simulink model "SVPWM_2L_Current_Loop"  (R2025a)
settings: Solver=VariableStepAuto  StartTime=0.0  StopTime=1  RelTol=1e-3
undefined symbols (not defined in the file): gTs
libraries: spsIGBTDiodeLib x6, spsVoltageMeasurementLib x6, spsACVoltageSourceLib x3, spsCurrentMeasurementLib x3, spsSeriesRLCBranchLib x3, simulink x1, spsDCVoltageSourceLib x1, sps_lib x1
settings Model: Creator=jicai  LastModifiedBy=jicai

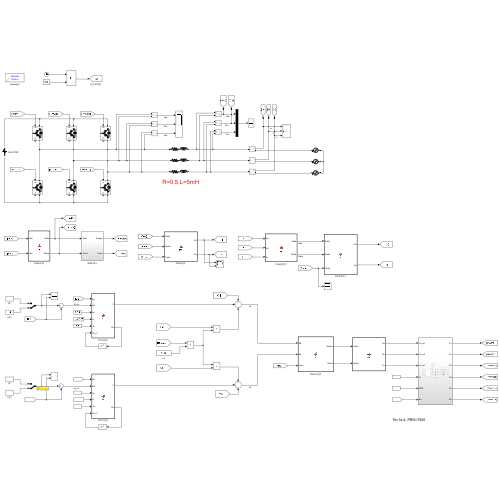
[thumbnail: Simulink's stored preview of the top-level diagram]
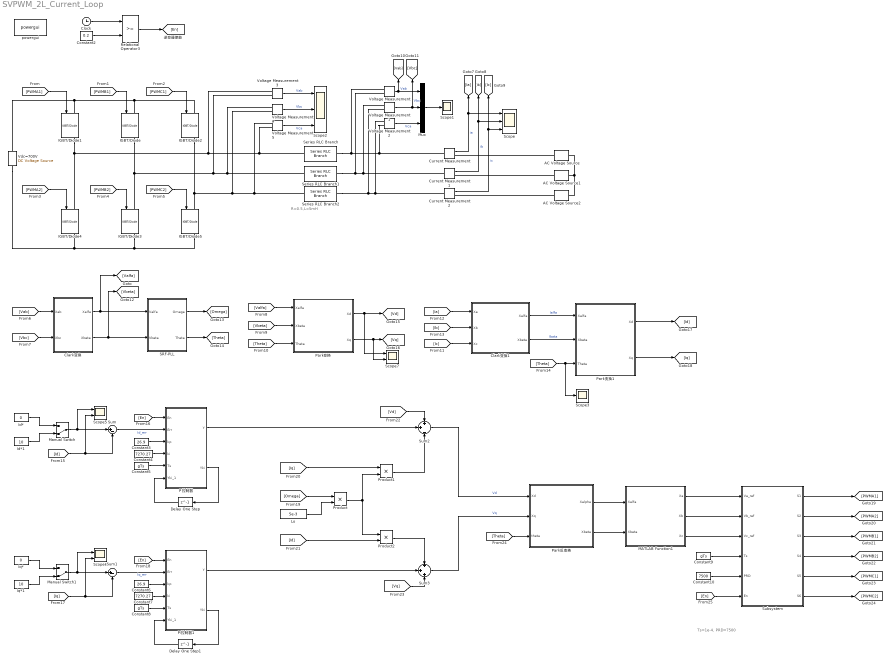
== system SVPWM_2L_Current_Loop ==
  note: R=0.5,L=5mH
  note: Ts=1e-4, PRD=7500
  AC Voltage Source : spsACVoltageSourceLib/AC Voltage Source  Amplitude=311  Phase=0  Frequency=50  SampleTime=1e-4  Measurements=None  BusType=swing  Pref=10e3  Qref=0  Qmin=-inf  Qmax=+inf
  AC Voltage Source1 : spsACVoltageSourceLib/AC Voltage Source  Amplitude=311  Phase=-120  Frequency=50  SampleTime=1e-4  Measurements=None  BusType=swing  Pref=10e3  Qref=0  Qmin=-inf  Qmax=+inf
  AC Voltage Source2 : spsACVoltageSourceLib/AC Voltage Source  Amplitude=311  Phase=120  Frequency=50  SampleTime=1e-4  Measurements=None  BusType=swing  Pref=10e3  Qref=0  Qmin=-inf  Qmax=+inf
  Clark变换 : MATLAB Function  TreatAsAtomicUnit=on
  Clark变换1 : MATLAB Function  TreatAsAtomicUnit=on
  Clock : Clock
  Constant10 : Constant  Value=7500
  Constant2 : Constant  Value=0.2
  Constant3 : Constant  Value=26.9
  Constant4 : Constant  Value=7270.27
  Constant5 : Constant  Value=gTs
  Constant6 : Constant  Value=26.9
  Constant7 : Constant  Value=7270.27
  Constant8 : Constant  Value=gTs
  Constant9 : Constant  Value=gTs
  Current Measurement : spsCurrentMeasurementLib/Current Measurement  PhasorSimulation=off  OutputType=Complex  PSBequivalent=0
  Current Measurement1 : spsCurrentMeasurementLib/Current Measurement  PhasorSimulation=off  OutputType=Complex  PSBequivalent=0
  Current Measurement2 : spsCurrentMeasurementLib/Current Measurement  PhasorSimulation=off  OutputType=Complex  PSBequivalent=0
  Delay One Step : Delay  DelayLength=1  SampleTime=1e-4
  Delay One Step1 : Delay  DelayLength=1  SampleTime=1e-4
  IGBT/Diode{,1..5} (6 alike) : spsIGBTDiodeLib/IGBT//Diode  Ron=1e-3  Rs=1e5  Cs=inf  Measurements=on
  Id* : Constant  Value=0
  Id*1 : Constant  Value=10
  Iq* : Constant  Value=0
  Iq*1 : Constant  Value=10
  Lo : Constant  Value=5e-3
  MATLAB Function1 : MATLAB Function  TreatAsAtomicUnit=on
  Manual Switch : ManualSwitch  CurrentSetting=0
  Manual Switch1 : ManualSwitch  CurrentSetting=0
  Mux : Mux  Inputs=3
  PI控制器 : MATLAB Function  TreatAsAtomicUnit=on
  PI控制器1 : MATLAB Function  TreatAsAtomicUnit=on
  Park反变换 : MATLAB Function  TreatAsAtomicUnit=on
  Park变换 : MATLAB Function  TreatAsAtomicUnit=on
  Park变换1 : MATLAB Function  TreatAsAtomicUnit=on
  Product : Product
  Product1 : Product
  Product2 : Product
  Relational Operator3 : RelationalOperator  OutDataTypeStr=boolean  RndMeth=Simplest  InputSameDT=off
  SRF-PLL : Subsystem
  Scope : Scope  NumInputPorts=3
      settings: ActiveDisplayYMinimum=-13.697929554868328  ActiveDisplayYMaximum=13.701744497418739
  Scope1 : Scope
      settings: ActiveDisplayYMinimum=-657.0084863452397  ActiveDisplayYMaximum=565.977190044395
  Scope2 : Scope  NumInputPorts=3
      settings: ActiveDisplayYMinimum=-1603.5172751574187  ActiveDisplayYMaximum=2906.9793668628458  DataLoggingVariableName=ScopeData2
  Scope3 : Scope
      settings: ActiveDisplayYMinimum=-0.78514945397904012  ActiveDisplayYMaximum=7.0684394809137565  DataLoggingVariableName=ScopeData3
  Scope5 : Scope  NumInputPorts=2
      settings: ActiveDisplayYMinimum=-0.80983118831991885  ActiveDisplayYMaximum=0.77229575693988206  DataLoggingVariableName=ScopeData5
  Scope6 : Scope  NumInputPorts=2
      settings: ActiveDisplayYMinimum=-2.4972295531085793  ActiveDisplayYMaximum=12.59917650103468  DataLoggingVariableName=ScopeData6
  Scope7 : Scope  NumInputPorts=2
      settings: ActiveDisplayYMinimum=-0.50666034266214766  ActiveDisplayYMaximum=8.8714736252296831  DataLoggingVariableName=ScopeData7
  Series RLC Branch : spsSeriesRLCBranchLib/Series RLC Branch  LConnTagsString=__new0  RConnTagsString=__new0  BranchType=RL  Resistance=0.5  Inductance=5e-3  SetiL0=off  InitialCurrent=0  Capacitance=1e-6  Setx0=off  InitialVoltage=0  Measurements=None
  Series RLC Branch1 : spsSeriesRLCBranchLib/Series RLC Branch  LConnTagsString=__new0  RConnTagsString=__new0  BranchType=RL  Resistance=0.5  Inductance=5e-3  SetiL0=off  InitialCurrent=0  Capacitance=1e-6  Setx0=off  InitialVoltage=0  Measurements=None
  Series RLC Branch2 : spsSeriesRLCBranchLib/Series RLC Branch  LConnTagsString=__new0  RConnTagsString=__new0  BranchType=RL  Resistance=0.5  Inductance=5e-3  SetiL0=off  InitialCurrent=0  Capacitance=1e-6  Setx0=off  InitialVoltage=0  Measurements=None
  Subsystem : Subsystem
  Sum : Sum  Inputs=|+-
  Sum1 : Sum  Inputs=|+-
  Sum2 : Sum  Inputs=+|+|-
  Sum3 : Sum  Inputs=+|+|+
  Vdc=700V : spsDCVoltageSourceLib/DC Voltage Source  Amplitude=700  Measurements=None
  Voltage Measurement{,1..5} (6 alike) : spsVoltageMeasurementLib/Voltage Measurement  PhasorSimulation=off  OutputType=Complex  PSBequivalent=0
  powergui : sps_lib/powergui  Priority=1  SimulationMode=Discrete  SampleTime=1e-6  frequency=60  Iterations=50  frequencyindice=0  Pbase=100e6  ErrMax=1e-4  UnitsV=kV  UnitsW=MW  buscounter=0  FunctionMessages=off  echomessages=off  EnableUseOfTLC=off  CurrentSourceSwitches=off  DisableSnubberDevices=off  DisableRonSwitches=off  DisableVfSwitches=off  DisplayEquations=off  AutomaticDiscreteSolvers=off  SolverType=Tustin/Backward Euler (TBE)  Interpol=off  ExternalGateDelay=off  methode=off  Ts=100  x0status=blocks  SPID=on  SwTol=0  HookPort=off  NonlinearTolerance=1e-4  nMaxIteration=100  ContinueOnMaxIteration=off  RestoreLinks=warning  ResistiveCurrentMeasurement=off  Frange=[0:2:500]  Ylog=off  Xlog=on  ShowGrid=off  save=off  variable=ZData  structure=0  ZoomFFT=off  StartTime=0.0  cycles=1  DisplayStyle=1  fundamental=60  FreqAxis=off  MaxFrequency=1000  frequencyindicesteady=1  RmsSteady=1  display=off
  wires:
  Current Measurement/1 -> Scope/1, [Ia]  "ia"
  Current Measurement1/1 -> Scope/2, [Ib]  "ib"
  Current Measurement2/1 -> [Ic], Scope/3  "ic"
  Voltage Measurement/1 -> [Vab], Mux/1  "Vab"
  Voltage Measurement1/1 -> [Vbc], Mux/2  "Vbc"
  Voltage Measurement2/1 -> Mux/3  "Vca"
  Mux/1 -> Scope1/1
  Voltage Measurement5/1 -> Scope2/3  "Vca"
  Voltage Measurement4/1 -> Scope2/2  "Vbc"
  Voltage Measurement3/1 -> Scope2/1  "Vab"
  [PWMA1] -> IGBT/Diode1/1
  [PWMB1] -> IGBT/Diode/1
  [PWMC1] -> IGBT/Diode2/1
  [PWMB2] -> IGBT/Diode3/1
  [PWMA2] -> IGBT/Diode4/1
  [PWMC2] -> IGBT/Diode5/1
  [Vab] -> Clark变换/1(Xab)
  [Vbc] -> Clark变换/2(Xbc)
  Clark变换/1(Xalfa) -> [Valfa], SRF-PLL/1(Valfa)
  Clark变换/2(Xbeta) -> [Vbeta], SRF-PLL/2(Vbeta)
  [Valfa] -> Park变换/1(Xalfa)
  [Vbeta] -> Park变换/2(Xbeta)
  [Theta] -> Park变换/3(Theta)
  Park变换/1(Xd) -> Scope7/1, [Vd]
  Park变换/2(Xq) -> Scope7/2, [Vq]
  [Ia] -> Clark变换1/1(Xa)
  [Ib] -> Clark变换1/2(Xb)
  [Ic] -> Clark变换1/3(Xc)
  Clark变换1/2(Xbeta) -> Park变换1/2(Xbeta)  "Ibata"
  Clark变换1/1(Xalfa) -> Park变换1/1(Xalfa)  "Ialfa"
  [Theta] -> Scope3/1, Park变换1/3(Theta)
  Park变换1/1(Xd) -> [Id]
  Park变换1/2(Xq) -> [Iq]
  Clock/1 -> Relational Operator3/1
  Constant2/1 -> Relational Operator3/2
  Relational Operator3/1 -> [En]
  Id*/1 -> Manual Switch/1
  Id*1/1 -> Manual Switch/2
  Manual Switch/1 -> Scope5/1, Sum/1
  [Id] -> Scope5/2, Sum/2
  [En] -> PI控制器/1(En)
  Sum/1 -> PI控制器/2(Err)  "Id_err"
  Constant3/1 -> PI控制器/3(kp)
  Constant4/1 -> PI控制器/4(ki)
  Constant5/1 -> PI控制器/5(Ts)
  PI控制器/2(Yki) -> Delay One Step/1
  Delay One Step/1 -> PI控制器/6(Yki_1)
  Delay One Step1/1 -> PI控制器1/6(Yki_1)
  PI控制器1/2(Yki) -> Delay One Step1/1
  Constant8/1 -> PI控制器1/5(Ts)
  Constant7/1 -> PI控制器1/4(ki)
  Constant6/1 -> PI控制器1/3(kp)
  Sum1/1 -> PI控制器1/2(Err)  "Iq_err"
  [En] -> PI控制器1/1(En)
  [Iq] -> Sum1/2, Scope6/2
  Manual Switch1/1 -> Sum1/1, Scope6/1
  Iq*1/1 -> Manual Switch1/2
  Iq*/1 -> Manual Switch1/1
  [Omega] -> Product/1
  Lo/1 -> Product/2
  Product/1 -> Product1/2, Product2/1
  [Iq] -> Product1/1
  [Id] -> Product2/2
  PI控制器/1(Y) -> Sum2/2
  [Vd] -> Sum2/1
  Product1/1 -> Sum2/3
  PI控制器1/1(Y) -> Sum3/2
  [Vq] -> Sum3/3
  Product2/1 -> Sum3/1
  [Theta] -> Park反变换/3(theta)
  Sum2/1 -> Park反变换/1(Xd)  "Vd"
  Sum3/1 -> Park反变换/2(Xq)  "Vq"
  Park反变换/1(Xalpha) -> MATLAB Function1/1(Xalfa)
  Park反变换/2(Xbeta) -> MATLAB Function1/2(Xbeta)
  [En] -> Subsystem/6(En)
  Subsystem/1(S1) -> [PWMA1]
  Subsystem/2(S2) -> [PWMA2]
  Subsystem/3(S3) -> [PWMB1]
  Subsystem/4(S4) -> [PWMB2]
  Subsystem/5(S5) -> [PWMC1]
  Subsystem/6(S6) -> [PWMC2]
  MATLAB Function1/3(Xc) -> Subsystem/3(Vc_ref)
  MATLAB Function1/1(Xa) -> Subsystem/1(Va_ref)
  MATLAB Function1/2(Xb) -> Subsystem/2(Vb_ref)
  Constant9/1 -> Subsystem/4(Ts)
  Constant10/1 -> Subsystem/5(PRD)
  SRF-PLL/1(Omega) -> [Omega]
  SRF-PLL/2(Theta) -> [Theta]
  connections:
  Vdc=700V/RConn1 -- IGBT/Diode1/LConn1 -- IGBT/Diode/LConn1 -- IGBT/Diode2/LConn1
  IGBT/Diode1/RConn1 -- Voltage Measurement3/LConn1 -- Voltage Measurement5/LConn2 -- Series RLC Branch/LConn1 -- IGBT/Diode4/LConn1
  IGBT/Diode/RConn1 -- Voltage Measurement4/LConn1 -- Series RLC Branch1/LConn1 -- Voltage Measurement3/LConn2 -- IGBT/Diode3/LConn1
  IGBT/Diode2/RConn1 -- Voltage Measurement4/LConn2 -- Voltage Measurement5/LConn1 -- Series RLC Branch2/LConn1 -- IGBT/Diode5/LConn1
  Vdc=700V/LConn1 -- IGBT/Diode4/RConn1 -- IGBT/Diode3/RConn1 -- IGBT/Diode5/RConn1
  Series RLC Branch/RConn1 -- Voltage Measurement/LConn1 -- Voltage Measurement2/LConn2 -- Current Measurement/LConn1
  Series RLC Branch1/RConn1 -- Voltage Measurement/LConn2 -- Voltage Measurement1/LConn1 -- Current Measurement1/LConn1
  Series RLC Branch2/RConn1 -- Voltage Measurement1/LConn2 -- Voltage Measurement2/LConn1 -- Current Measurement2/LConn1
  AC Voltage Source1/LConn1 -- AC Voltage Source2/LConn1 -- AC Voltage Source/LConn1
  AC Voltage Source/RConn1 -- Current Measurement/RConn1
  AC Voltage Source1/RConn1 -- Current Measurement1/RConn1
  AC Voltage Source2/RConn1 -- Current Measurement2/RConn1

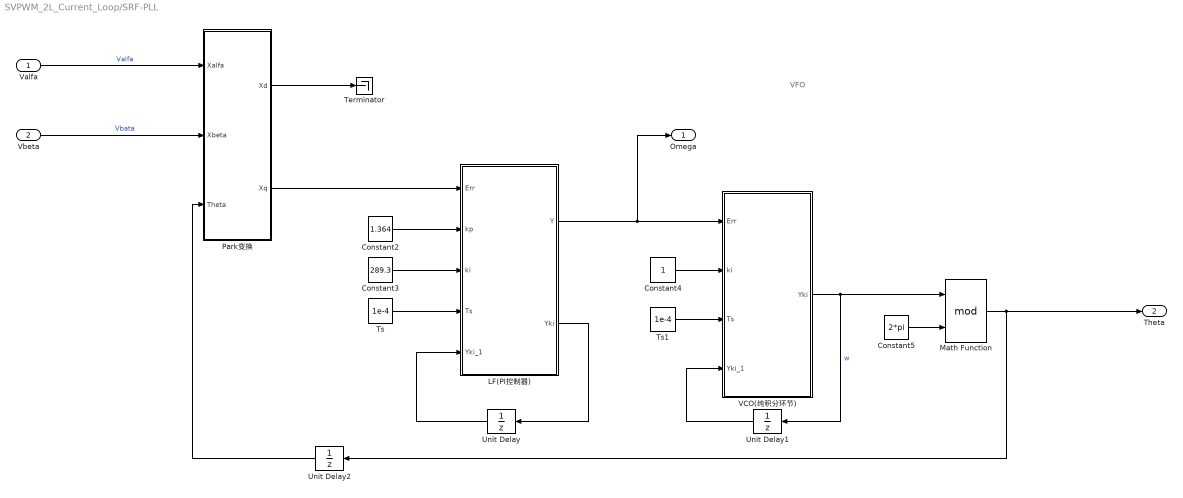
== system SVPWM_2L_Current_Loop/SRF-PLL ==
  note: VFO
  Valfa : Inport
  Vbeta : Inport  Port=2
  Constant2 : Constant  Value=1.364
  Constant3 : Constant  Value=289.3
  Constant4 : Constant
  Constant5 : Constant  Value=2*pi
  LF(PI控制器) : MATLAB Function  TreatAsAtomicUnit=on
  Math Function : Math  Operator=mod
  Park变换 : MATLAB Function  TreatAsAtomicUnit=on
  Terminator : Terminator
  Ts : Constant  Value=1e-4
  Ts1 : Constant  Value=1e-4
  Unit Delay : UnitDelay  SampleTime=1e-4  HasFrameUpgradeWarning=on
  Unit Delay1 : UnitDelay  SampleTime=1e-4  HasFrameUpgradeWarning=on
  Unit Delay2 : UnitDelay  SampleTime=1e-4  HasFrameUpgradeWarning=on
  VCO(纯积分环节) : MATLAB Function  TreatAsAtomicUnit=on
  Omega : Outport
  Theta : Outport  Port=2
  wires:
  Constant5/1 -> Math Function/2
  Math Function/1 -> Theta/1, Unit Delay2/1
  Vbeta/1 -> Park变换/2(Xbeta)  "Vbata"
  VCO(纯积分环节)/1(Yki) -> Unit Delay1/1, Math Function/1  "w"
  Constant3/1 -> LF(PI控制器)/3(ki)
  Park变换/2(Xq) -> LF(PI控制器)/1(Err)
  Constant2/1 -> LF(PI控制器)/2(kp)
  Valfa/1 -> Park变换/1(Xalfa)  "Valfa"
  Constant4/1 -> VCO(纯积分环节)/2(ki)
  Unit Delay/1 -> LF(PI控制器)/5(Yki_1)
  Park变换/1(Xd) -> Terminator/1
  Unit Delay2/1 -> Park变换/3(Theta)
  LF(PI控制器)/1(Y) -> Omega/1, VCO(纯积分环节)/1(Err)
  Ts/1 -> LF(PI控制器)/4(Ts)
  LF(PI控制器)/2(Yki) -> Unit Delay/1
  Unit Delay1/1 -> VCO(纯积分环节)/4(Yki_1)
  Ts1/1 -> VCO(纯积分环节)/3(Ts)

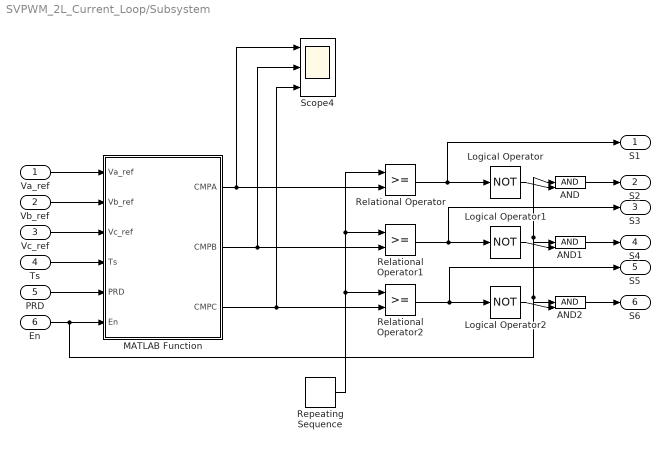
== system SVPWM_2L_Current_Loop/Subsystem ==
  Va_ref : Inport
  Vb_ref : Inport  Port=2
  Vc_ref : Inport  Port=3
  Ts : Inport  Port=4
  PRD : Inport  Port=5
  En : Inport  Port=6
  AND : Logic  IconShape=distinctive  AllPortsSameDT=off  OutDataTypeStr=boolean
  AND1 : Logic  IconShape=distinctive  AllPortsSameDT=off  OutDataTypeStr=boolean
  AND2 : Logic  IconShape=distinctive  AllPortsSameDT=off  OutDataTypeStr=boolean
  Logical Operator : Logic  Operator=NOT  AllPortsSameDT=off  OutDataTypeStr=boolean
  Logical Operator1 : Logic  Operator=NOT  AllPortsSameDT=off  OutDataTypeStr=boolean
  Logical Operator2 : Logic  Operator=NOT  AllPortsSameDT=off  OutDataTypeStr=boolean
  MATLAB Function : MATLAB Function  TreatAsAtomicUnit=on
  Relational Operator : RelationalOperator  OutDataTypeStr=boolean  RndMeth=Simplest  InputSameDT=off
  Relational Operator1 : RelationalOperator  OutDataTypeStr=boolean  RndMeth=Simplest  InputSameDT=off
  Relational Operator2 : RelationalOperator  OutDataTypeStr=boolean  RndMeth=Simplest  InputSameDT=off
  Repeating Sequence : simulink/Sources/Repeating Sequence  rep_seq_t=[0 5e-5 1e-4]  rep_seq_y=[0 7500 0]
  Scope4 : Scope  NumInputPorts=3
      settings: ActiveDisplayYMinimum=-937.5  ActiveDisplayYMaximum=8437.5000000000018  DataLoggingVariableName=ScopeData4
  S1 : Outport
  S2 : Outport  Port=2
  S3 : Outport  Port=3
  S4 : Outport  Port=4
  S5 : Outport  Port=5
  S6 : Outport  Port=6
  wires:
  Relational Operator2/1 -> S5/1, Logical Operator2/1
  MATLAB Function/1(CMPA) -> Scope4/1, Relational Operator/2
  Relational Operator/1 -> S1/1, Logical Operator/1
  MATLAB Function/3(CMPC) -> Scope4/3, Relational Operator2/2
  Relational Operator1/1 -> S3/1, Logical Operator1/1
  MATLAB Function/2(CMPB) -> Scope4/2, Relational Operator1/2
  Repeating Sequence/1 -> Relational Operator/1, Relational Operator1/1, Relational Operator2/1
  Va_ref/1 -> MATLAB Function/1(Va_ref)
  En/1 -> AND1/1, AND/1, AND2/1, MATLAB Function/6(En)
  Vb_ref/1 -> MATLAB Function/2(Vb_ref)
  Vc_ref/1 -> MATLAB Function/3(Vc_ref)
  Ts/1 -> MATLAB Function/4(Ts)
  PRD/1 -> MATLAB Function/5(PRD)
  AND/1 -> S2/1
  Logical Operator/1 -> AND/2
  Logical Operator1/1 -> AND1/2
  AND1/1 -> S4/1
  Logical Operator2/1 -> AND2/2
  AND2/1 -> S6/1

== matlab function SVPWM_2L_Current_Loop/PI控制器1 ==
  data: En input; Err input; Y output; kp input; ki input; Yki output; Ts input; Yki_1 input
function [Y, Yki] = PI(En, Err, kp, ki, Ts, Yki_1)

% 采用的离散化方法： s = (1-z^{-1})/Ts

max = 3000;  % 限幅
min = -3000;

% 计算积分项
Yki = Yki_1 + Ts*ki*Err;
if Yki > max
    Yki = max;
elseif Yki < min
    Yki = min;
end

% 加上比例项
if En == 1
    Y = kp*Err + Yki;
else
    Y = 0;
    Yki = 0;
end

if Y > max
    Y = max;
elseif Y < min
    Y = min;
end
end

== matlab function SVPWM_2L_Current_Loop/Park反变换 ==
  data: Xd input; Xalpha output; Xq input; theta input; Xbeta output
function [Xalpha, Xbeta] = fcn(Xd, Xq, theta)
% 该函数实现 Park 反变换：从旋转坐标系 (dq) 转换到静止坐标系 (alpha-beta)
% 输入参数：
% Xd    - d轴分量
% Xq    - q轴分量
% theta - 旋转电角度（弧度）

% 根据坐标变换公式：
% Xalpha = Xd * cos(theta) - Xq * sin(theta)
% Xbeta  = Xd * sin(theta) + Xq * cos(theta)

Xalpha = Xd * cos(theta) - Xq * sin(theta);
Xbeta  = Xd * sin(theta) + Xq * cos(theta);

== matlab function SVPWM_2L_Current_Loop/MATLAB Function1 ==
  data: Xalfa input; Xa output; Xbeta input; Xb output; Xc output
function [Xa, Xb, Xc] = fcn(Xalfa, Xbeta)
% 该函数实现 Clarke 反变换：从 alpha-beta 坐标系转换回 abc 三相坐标系
% 基于等幅值变换原则

% 根据逆矩阵推导：
% Xa = Xalfa
% Xb = -0.5 * Xalfa + sqrt(3)/2 * Xbeta
% Xc = -0.5 * Xalfa - sqrt(3)/2 * Xbeta

Xa = Xalfa;
Xb = -0.5 * Xalfa + (sqrt(3)/2) * Xbeta;
Xc = -0.5 * Xalfa - (sqrt(3)/2) * Xbeta;

== matlab function SVPWM_2L_Current_Loop/Clark变换 ==
  data: Xab input; Xalfa output; Xbc input; Xbeta output
%由 $V_{ab},V_{bc}$ 转换为 $V_{alfa},V_{beta}$ 的Clark变换：

function[Xalfa,Xbeta] =fcn(Xab,Xbc)
% Xalfa = 2/3*(Xa - 0.5*Xb - 0.5*Xc);
%       = 2/3*(Xa -Xb +(0.5*Xb - 0.5*Xc))
%       = 2/3*(Xab + 0.5*Xbc);

Xalfa = 2/3*(Xab + 0.5*Xbc);
Xbeta = sqrt(3)/3*Xbc;

== matlab function SVPWM_2L_Current_Loop/Subsystem/MATLAB Function ==
  data: Va_ref input; Vb_ref input; Vc_ref input; Ts input; PRD input; CMPA output; CMPB output; CMPC output; En input
function [CMPA,CMPB,CMPC] = SVPWM(Va_ref, Vb_ref, Vc_ref, Ts, PRD, En)

Va = Va_ref;
Vb = Vb_ref;
Vc = Vc_ref;
Ts = Ts;
PRD = PRD;
EN = En;


%% 60°坐标变换

Vg = 2/3 * (Va - Vb);
Vh = 2/3 * (Vb - Vc);

% 进行标幺化
Vdc = 700;
Vg = Vg/(2*Vdc/3);
Vh = Vh/(2*Vdc/3);

%% 判断扇区、 其他扇区与第1扇区的映射关系

if(Vh>=0 && Vg>=0)
    Sec = 1;
    Vgg = Vg;
    Vhh = Vh;
elseif(Vh>=0 && Vg+Vh>=0)
    Sec = 2;
    Vhh = Vg + Vh;   % 注意第2、4、6扇区 的起始矢量顺序，与第1扇区的区别
    Vgg = -Vg;
elseif(Vh>=0 && Vg+Vh<=0)
    Sec = 3;
    Vgg = Vh;
    Vhh = -Vg - Vh;
elseif(Vg<=0 && Vh<=0)
    Sec = 4;
    Vhh = -Vg;
    Vgg = -Vh;
elseif(Vg>=0 && Vg+Vh<=0)
    Sec = 5;
    Vgg = -Vg - Vh;
    Vhh = Vg;
else
    Sec = 6;
    Vhh = -Vh;
    Vgg = Vg + Vh;
end


%% 计算 T0、T1、T2矢量的作用时间
T1 = Vgg;    % 这里本来应该乘以 Ts，但是在下面计算CL时，又要除以Ts，
T2 = Vhh;    % 因此，可以同时省去。
T0 = 1- T1 - T2;

if (T0 < 0)
    Tsum = T1 + T2;
    T1 = T1/Tsum;
    T2 = T2/Tsum;
    T0 = 0;
end
    
TL = 0.25 * T0;
TM = TL + 0.5 * T1;
TH = TM + 0.5 * T2;

CL = TL * PRD * 2;
CM = TM * PRD * 2;
CH = TH * PRD * 2;


%% 根据扇区，确定a、b、c三相CMP寄存器的值。

switch Sec
    case 1
        CMPA = CL;
        CMPB = CM;
        CMPC = CH;
    case 2
        CMPA = CM;
        CMPB = CL;
        CMPC = CH;
    case 3
        CMPA = CH;
        CMPB = CL;
        CMPC = CM;
    case 4
        CMPA = CH;
        CMPB = CM;
        CMPC = CL;
    case 5
        CMPA = CM;
        CMPB = CH;
        CMPC = CL;
    case 6
        CMPA = CL;
        CMPB = CH;
        CMPC = CM;
    otherwise 
        CMPA = CL;  % 不会进入这个分支，但是matlab要求必须有 otherwise
        CMPB = CH;
        CMPC = CM;    
end

if EN == 0
    CMPA = PRD;
    CMPB = PRD;
    CMPC = PRD;
end

== matlab function SVPWM_2L_Current_Loop/Park变换 ==
  data: Xalfa input; Xd output; Xbeta input; Theta input; Xq output
function [Xd,Xq] = fcn(Xalfa,Xbeta,Theta)
Xd = Xalfa * cos(Theta) + Xbeta * sin(Theta);
Xq = -Xalfa * sin(Theta) + Xbeta * cos(Theta);

== matlab function SVPWM_2L_Current_Loop/SRF-PLL/LF(PI控制器) ==
  data: Err input; Y output; kp input; ki input; Yki output; Ts input; Yki_1 input
function [Y, Yki] = PI(Err, kp, ki,Ts,Yki_1)

% 采用的离散化方法： s = (1-z^{-1})/Ts

max = 3000;  % 限幅
min = -3000;

% 计算积分项
Yki = Yki_1 + Ts*ki*Err;
if Yki > max
    Yki = max;
elseif Yki < min
    Yki = min;
end

% 加上比例项 
Y = kp*Err + Yki;

if Y > max
    Y = max;
elseif Y < min
    Y = min;
end
end

== matlab function SVPWM_2L_Current_Loop/SRF-PLL/Park变换 ==
  data: Xalfa input; Xd output; Xbeta input; Theta input; Xq output
function [Xd,Xq] = fcn(Xalfa,Xbeta,Theta)
Xd = Xalfa * cos(Theta) + Xbeta * sin(Theta);
Xq = -Xalfa * sin(Theta) + Xbeta * cos(Theta);

== matlab function SVPWM_2L_Current_Loop/SRF-PLL/VCO(纯积分环节) ==
  data: Err input; ki input; Yki output; Ts input; Yki_1 input
function Yki  = PI(Err, ki,Ts,Yki_1)

% 采用的离散化方法： s = (1-z^{-1})/Ts

max = 3000;
min = -3000;

% 计算积分项
Yki = Yki_1 + Ts*ki*Err;

if Yki > max
    Yki = max;
elseif Yki < min
    Yki = min;
end
end

== matlab function SVPWM_2L_Current_Loop/Clark变换1 ==
  data: Xa input; Xalfa output; Xb input; Xc input; Xbeta output
function [Xalfa,Xbeta] = fcn(Xa,Xb,Xc)
Xalfa = 2/3*(Xa - 0.5*Xb - 0.5*Xc);
Xbeta = sqrt(3)/3*(Xb-Xc);

== matlab function SVPWM_2L_Current_Loop/Park变换1 ==
  data: Xalfa input; Xd output; Xbeta input; Theta input; Xq output
function [Xd,Xq] = fcn(Xalfa,Xbeta,Theta)
Xd = Xalfa * cos(Theta) + Xbeta * sin(Theta);
Xq = -Xalfa * sin(Theta) + Xbeta * cos(Theta);

== matlab function SVPWM_2L_Current_Loop/PI控制器 ==
  data: En input; Err input; Y output; kp input; ki input; Yki output; Ts input; Yki_1 input
function [Y, Yki] = PI(En, Err, kp, ki,Ts,Yki_1)

% 采用的离散化方法： s = (1-z^{-1})/Ts

max = 3000;  % 限幅
min = -3000;

% 计算积分项
Yki = Yki_1 + Ts*ki*Err;
if Yki > max
    Yki = max;
elseif Yki < min
    Yki = min;
end

% 加上比例项
if En == 1
    Y = kp*Err + Yki;
else
    Y = 0;
    Yki = 0;
end

if Y > max
    Y = max;
elseif Y < min
    Y = min;
end
end
